simulink model "LQR_1"  (R2021b)
settings: Solver=VariableStepAuto  StartTime=0.0  StopTime=10.0  RelTol=1e-3
undefined symbols (not defined in the file): A, B, X0
libraries: dspinverses x1, dspmtrx3 x1
settings Model: Creator=nvnma  LastModifiedBy=nvnma

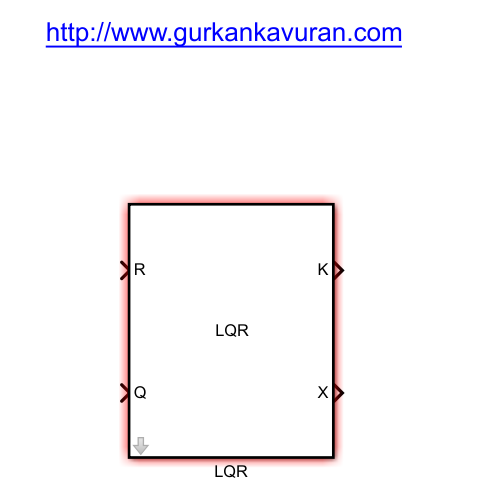
[thumbnail: Simulink's stored preview of the top-level diagram]
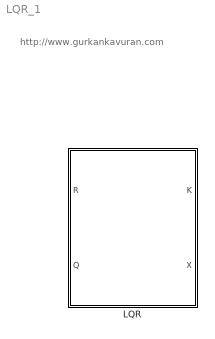
== system LQR_1 ==
  note: http://www.gurkankavuran.com
  LQR : Subsystem  Description=|  TreatAsAtomicUnit=on  mask(LQR with Algebric Riccati Equation){A=A, B=B, X0=X0}
      | LQR Block
      | 
      | by Gurkan KAVURAN
      | gurkankavuran@gmail.com
      mask prompts: A "A (System Matrix)"; B "B (System Matrix)"; X0 "Xo (Initial Values of States)"
      mask help:
      | It is easy to optimize Q and R matrices with online process.
      | Please see the help file to define the block parameters.
      mask Help:
      | Parameters Example:
      | 
      | Q = diag([500 1 1 0 1 1] );
      | R = 1*diag([0.01 0.01 0.01 0.01]);
      | X0=[0 0 0 0 0 0;0 0 0 0 0 0;0 0 0 0 0 0;0 0 0 0 0 0;0 0 0 0 0 0;0 0 0 0 0 0];
      | 
      | "Matrix multiply" block is recommended to use in state feedback control mechanism.
      | 
      | 
      | http://www.gurkankavuran.com
      mask Display:
      | disp('LQR')
      | port_label('input', 1, 'R')
      | port_label('input', 2, 'Q')
      | port_label('output', 1, 'K')
      | port_label('output', 2, 'X')

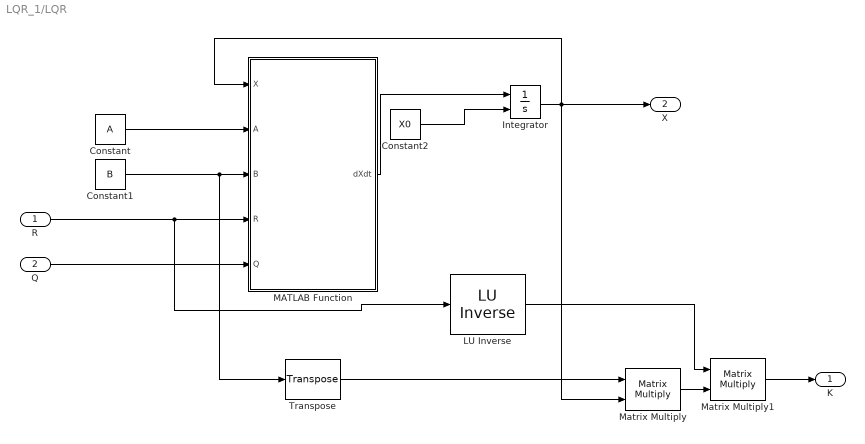
== system LQR_1/LQR ==
  R : Inport
  Q : Inport  Port=2
  " LU Inverse" : dspinverses/ LU Inverse
  Constant : Constant  Value=A
  Constant1 : Constant  Value=B
  Constant2 : Constant  Value=X0
  Integrator : Integrator  InitialConditionSource=external  InitialCondition=[1 1 1 1 1 1 1 1 1 1 1 1 1 1 1 1 1 1 1 1 1 1 1 1 1 1 1 1 1 1 1 1 1 1 1 1]
  MATLAB Function : MATLAB Function  TreatAsAtomicUnit=on
  Matrix Multiply : Product  Multiplication=Matrix(*)
  Matrix Multiply1 : Product  Multiplication=Matrix(*)
  Transpose : dspmtrx3/Transpose  Hermitian=off  overflowFlag=off
      settings: SourceProductBaseCode=DS
  K : Outport
  X : Outport  Port=2
  wires:
  Matrix Multiply1/1 -> K/1
  Constant/1 -> MATLAB Function/2(A)
  Constant1/1 -> Transpose/1, MATLAB Function/3(B)
  " LU Inverse"/1 -> Matrix Multiply1/1
  Constant2/1 -> Integrator/2
  Matrix Multiply/1 -> Matrix Multiply1/2
  Transpose/1 -> Matrix Multiply/1
  MATLAB Function/1(dXdt) -> Integrator/1
  Integrator/1 -> X/1, Matrix Multiply/2, MATLAB Function/1(X)
  Q/1 -> MATLAB Function/5(Q)
  R/1 -> " LU Inverse"/1, MATLAB Function/4(R)

== matlab function LQR_1/LQR/MATLAB Function ==
  data: dXdt output; X input; A input; B input; R input; Q input
function dXdt  = mRiccati(X, A, B,R,Q)
% r1=randi([1 1000]);
% r2=randi([1 1000]);
% r3=randi([1 1000]);
% r4=randi([1 1000]);
% r5=randi([1 1000]);
% r6=randi([1 1000]);
% Q = diag([r1 r2 r3 r4 r5 r6] );
% R = 1*diag([1 1 1 1]);
X = reshape(X, size(A)); %Convert from "n^2"-by-1 to "n"-by-"n"
dXdt = A.'*X + X*A - (X*B)*inv(R)*(B.'*X) + Q; %Determine derivative
% dXdtS= dXdt(:); %Convert from "n"-by-"n" to "n^2"-by-1,algebraic Riccati equation (ARE)
